simulink model "thermal_electrical"  (R2019b)
settings: Solver=VariableStepAuto  StartTime=0.0  StopTime=10.0  RelTol=1e-3
settings Model: Creator=aksha  LastModifiedBy=aksha

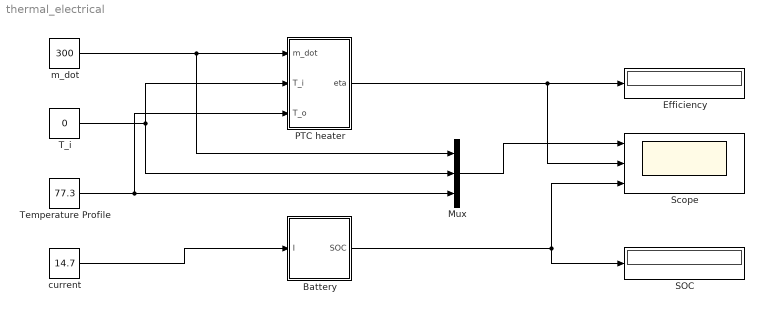
== system thermal_electrical ==
  Battery : Subsystem
  Efficiency : Display
  Mux : Mux  Inputs=3
  PTC heater : Subsystem
  SOC : Display
      settings: Decimation=4
  Scope : Scope  NumInputPorts=3
  T_i : Constant  Value=0
  Temperature Profile : Constant  Value=77.3
  current : Constant  Value=14.7
  m_dot : Constant  Value=300
  wires:
  m_dot/1 -> Mux/1, PTC heater/1(m_dot)
  T_i/1 -> PTC heater/2(T_i), Mux/2
  Temperature Profile/1 -> PTC heater/3(T_o), Mux/3
  PTC heater/1(eta) -> Scope/2, Efficiency/1
  Mux/1 -> Scope/1
  Battery/1(SOC) -> SOC/1, Scope/3
  current/1 -> Battery/1(I)

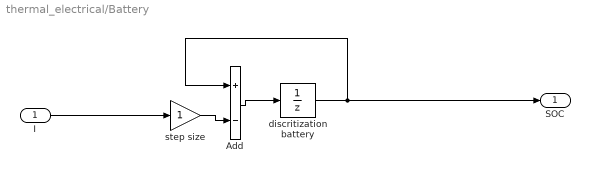
== system thermal_electrical/Battery ==
  I : Inport
  Add : Sum  Inputs=+-
  discritization battery : UnitDelay  InitialCondition=18000  HasFrameUpgradeWarning=on
  step size : Gain
  SOC : Outport
  wires:
  I/1 -> step size/1
  step size/1 -> Add/2
  discritization battery/1 -> SOC/1, Add/1
  Add/1 -> discritization battery/1

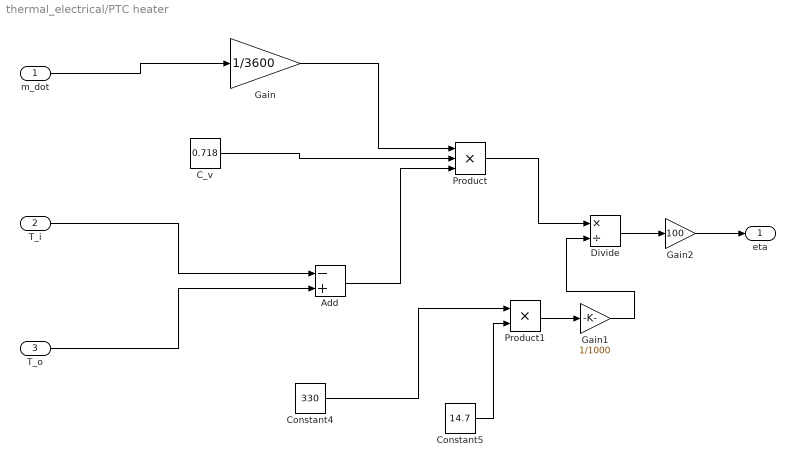
== system thermal_electrical/PTC heater ==
  m_dot : Inport
  T_i : Inport  Port=2
  T_o : Inport  Port=3
  Add : Sum  Inputs=-+
  C_v : Constant  Value=0.718
  Constant4 : Constant  Value=330
  Constant5 : Constant  Value=14.7
  Divide : Product  Inputs=*/
  Gain : Gain  Gain=1/3600
  Gain1 : Gain  Gain=1/1000
  Gain2 : Gain  Gain=100
  Product : Product  Inputs=3
  Product1 : Product
  eta : Outport
  wires:
  Gain/1 -> Product/1
  Product1/1 -> Gain1/1
  Add/1 -> Product/3
  Constant4/1 -> Product1/1
  Gain1/1 -> Divide/2
  Product/1 -> Divide/1
  Constant5/1 -> Product1/2
  C_v/1 -> Product/2
  T_i/1 -> Add/1
  T_o/1 -> Add/2
  m_dot/1 -> Gain/1
  Divide/1 -> Gain2/1
  Gain2/1 -> eta/1
